simulink model "final_10_7_23_simulink"  (R2021a)
settings: Solver=ode4  StartTime=0.0  StopTime=10.0  FixedStep=0.0001  RelTol=1e-3
libraries: cstblocks x1
settings Model: Creator=aghersin  LastModifiedBy=pedro
settings SolverCC: AlgebraicLoopSolver=TrustRegion
settings DataIOCC: ReturnWorkspaceOutputs=off
settings OptimizationCC: LifeSpan=inf
settings DebuggingCC: SFExecutionAtInitializationDiag=none  SFMachineParentedDataDiag=warning  ArithmeticOperatorsInVariantConditions=warning
settings SFSimCC: SimUseLocalCustomCode=off  CustomCodeUndefinedFunction=UseInterfaceOnly
settings RTWCC: RTWUseLocalCustomCode=off
settings CodeAppCC: StateflowObjectComments=on

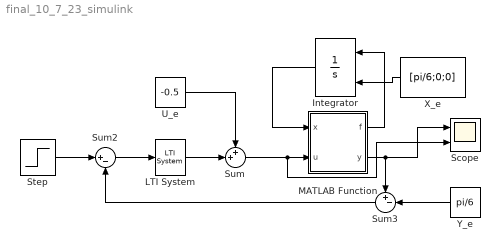
== system final_10_7_23_simulink ==
  Integrator : Integrator  InitialConditionSource=external
  LTI System : cstblocks/LTI System  sys=c_digital  IC=[]
  MATLAB Function : MATLAB Function  TreatAsAtomicUnit=on
  Scope : Scope  NumInputPorts=2
  Step : Step  After=2*180/pi  SampleTime=0
  Sum : Sum  Inputs=++|
  Sum2 : Sum  Inputs=|+-
  Sum3 : Sum  Inputs=+-|
  U_e : Constant  Value=-0.5
  X_e : Constant  Value=[pi/6;0;0]
  Y_e : Constant  Value=pi/6
  wires:
  Integrator/1 -> MATLAB Function/1(x)
  MATLAB Function/1(f) -> Integrator/1
  X_e/1 -> Integrator/2
  MATLAB Function/2(y) -> Sum3/1, Scope/1
  Y_e/1 -> Sum3/2
  U_e/1 -> Sum/1
  Sum2/1 -> LTI System/1
  Step/1 -> Sum2/1
  Sum3/1 -> Sum2/2
  LTI System/1 -> Sum/2
  Sum/1 -> Scope/2, MATLAB Function/2(u)

== matlab function final_10_7_23_simulink/MATLAB Function ==
  data: x input; u input; f output; y output
function [f,y] = fcn(x,u)
%constantes
p=4;

%f es mi X_punto
f1 = x(2);
f2 = sin(x(1)-0.1*x(2)+x(3));
f3 = p*(u-x(3));

f = [f1;f2;f3];

y=x(1);
